simulink model "mux_FM_mod_demod"  (R2023b)
settings: Solver=VariableStepAuto  StartTime=0.0  StopTime=2  RelTol=1e-3
undefined symbols (not defined in the file): fc1_mux, fc2_mux, fc3_mux, fm1_mux, fm2_mux, fm3_mux, ts_mux
libraries: commanapbnd3 x2
settings Model: Creator=RomaW11  LastModifiedBy=RomaW11

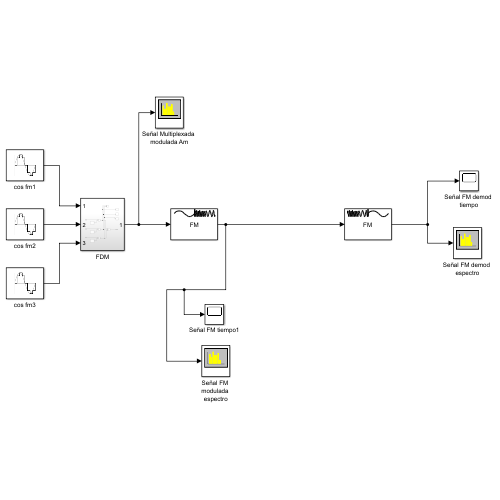
[thumbnail: Simulink's stored preview of the top-level diagram]
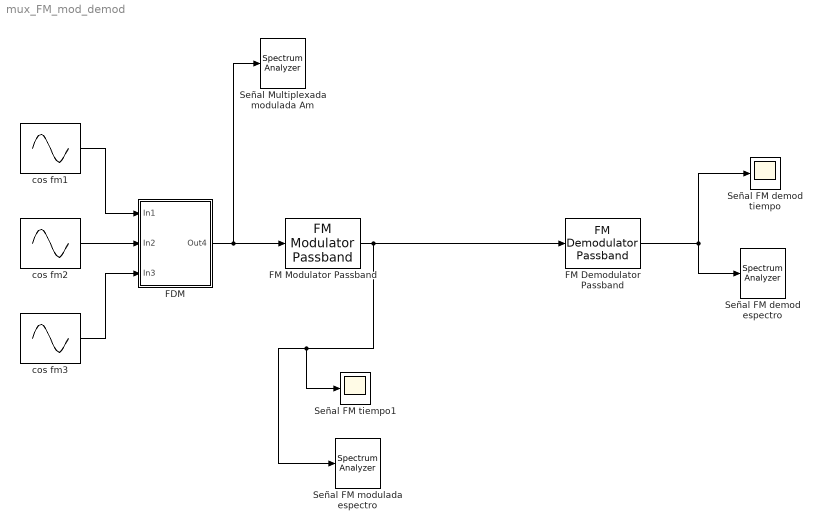
== system mux_FM_mod_demod ==
  FDM : Subsystem
  FM Demodulator Passband : commanapbnd3/FM Demodulator Passband  Fc=fc_mod_fm  Ph=0  Kc=50  Ho=100
  FM Modulator Passband : commanapbnd3/FM Modulator Passband  Fc=fc_mod_fm  Ph=0  Kc=50
  Señal FM modulada espectro : SpectrumAnalyzer  WindowPosition=[1.000000,1.000000,1920.000000,1057.000000,]  ScopeFrameLocation=window  SampleRate=44.1e3  StartFrequency=20  StopFrequency=20e3  YLimits=[-246.88599121,53.29540529]  ShowLegend=on
      settings: OpenAtSimulationStart=off
  Señal FM demod espectro : SpectrumAnalyzer  WindowPosition=[1.000000,1.000000,1920.000000,1057.000000,]  ScopeFrameLocation=window  SampleRate=44.1e3  StartFrequency=20  StopFrequency=20e3  YLimits=[-69.60389106,27.43586964]  ShowLegend=on
      settings: OpenAtSimulationStart=off
  Señal FM demod tiempo : Scope
  Señal FM tiempo1 : Scope
  Señal Multiplexada modulada Am : SpectrumAnalyzer  WindowPosition=[1.000000,1.000000,1920.000000,1057.000000,]  ScopeFrameLocation=window  SampleRate=44.1e3  StartFrequency=20  StopFrequency=20e3  Title=Señal modulada Am Multiplexada  YLimits=[-54.57593285,25.7705198]  ShowLegend=on
      settings: OpenAtSimulationStart=off
  cos fm1 : Sin  Frequency=2*pi*fm1_mux  Phase=pi/2  SampleTime=ts_mux
  cos fm2 : Sin  Frequency=2*pi*fm2_mux  Phase=pi/2  SampleTime=ts_mux
  cos fm3 : Sin  Frequency=2*pi*fm3_mux  Phase=pi/2  SampleTime=ts_mux
  wires:
  FDM/1(Out4) -> FM Modulator Passband/1, Señal Multiplexada modulada Am/1
  cos fm1/1 -> FDM/1(In1)
  cos fm2/1 -> FDM/2(In2)
  cos fm3/1 -> FDM/3(In3)
  FM Demodulator Passband/1 -> Señal FM demod espectro/1, Señal FM demod tiempo/1
  FM Modulator Passband/1 -> FM Demodulator Passband/1, Señal FM modulada espectro/1, Señal FM tiempo1/1

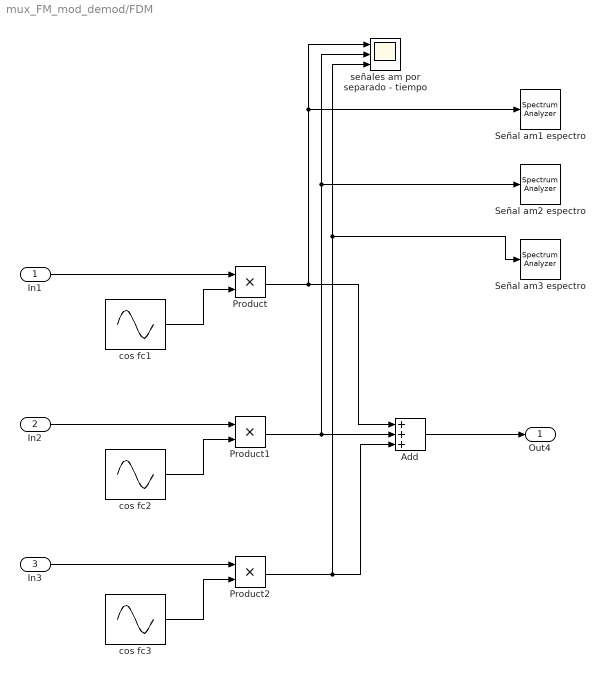
== system mux_FM_mod_demod/FDM ==
  In1 : Inport
  In2 : Inport  Port=2
  In3 : Inport  Port=3
  Add : Sum  Inputs=+++
  Product : Product
  Product1 : Product
  Product2 : Product
  Señal am1 espectro : SpectrumAnalyzer  WindowPosition=[1.000000,1.000000,1920.000000,1057.000000,]  ScopeFrameLocation=window  SampleRate=44.1e3  StartFrequency=20  StopFrequency=20e3  YLimits=[-65.29745179,26.83993796]  ShowLegend=on
      settings: OpenAtSimulationStart=off
  Señal am2 espectro : SpectrumAnalyzer  WindowPosition=[1.000000,1.000000,1920.000000,1057.000000,]  ScopeFrameLocation=window  SampleRate=44.1e3  StartFrequency=20  StopFrequency=20e3  YLimits=[-65.31113844,26.96311882]  ShowLegend=on
      settings: OpenAtSimulationStart=off
  Señal am3 espectro : SpectrumAnalyzer  WindowPosition=[1.000000,1.000000,1920.000000,1057.000000,]  ScopeFrameLocation=window  SampleRate=44.1e3  StartFrequency=20  StopFrequency=20e3  YLimits=[-65.31099224,26.96180511]  ShowLegend=on  ExpandToolstrip=on
      settings: OpenAtSimulationStart=off
  cos fc1 : Sin  Frequency=2*pi*fc1_mux  Phase=pi/2  SampleTime=ts_mux
  cos fc2 : Sin  Frequency=2*pi*fc2_mux  Phase=pi/2  SampleTime=ts_mux
  cos fc3 : Sin  Frequency=2*pi*fc3_mux  Phase=pi/2  SampleTime=ts_mux
  señales am por separado - tiempo : Scope  NumInputPorts=3
  Out4 : Outport
  wires:
  cos fc3/1 -> Product2/2
  Product2/1 -> señales am por separado - tiempo/3, Señal am3 espectro/1, Add/3
  cos fc2/1 -> Product1/2
  In1/1 -> Product/1
  In2/1 -> Product1/1
  Product/1 -> Señal am1 espectro/1, señales am por separado - tiempo/1, Add/1
  Product1/1 -> Señal am2 espectro/1, señales am por separado - tiempo/2, Add/2
  cos fc1/1 -> Product/2
  In3/1 -> Product2/1
  Add/1 -> Out4/1
